simulink model "simTr"  (R2018b)
settings: Solver=FixedStepAuto  StartTime=0.0  StopTime=100  FixedStep=0.001  RelTol=1e-3
values from neighbouring files (symbols this model uses):
  dfwe1 = 0.1 * fwe1max    [script8.m]
  dt = 20    [script8.m]
  fwe2 = 0.2594    [script8.m]
  h10 = (fwe1 / a1) + h20    [script8.m]
  h20 = (fwe1 + fwe2)/a2    [script8.m]
  Lh1f1 = [A2 a1+a2]    [script8.m]
  Lh1f2 = [a1]    [script8.m]
  Lh2f1 = [a1]    [script8.m]
  Lh2f2 = [A1 a1]    [script8.m]
  M = [A1*A2 a1*A1+a2*A1+a1*A2 a1*a1+a1*a2]    [script8.m]
settings Model: Creator=wojciechkonury  LastModifiedBy=wojciechkonury

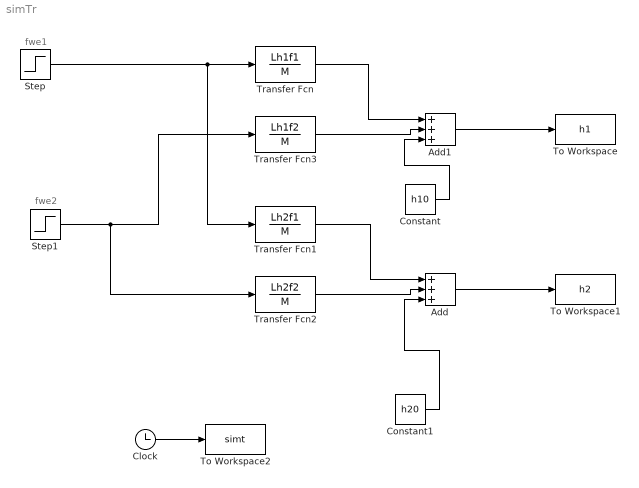
== system simTr ==
  note: fwe2
  note: fwe1
  Add : Sum  Inputs=+++
  Add1 : Sum  Inputs=+++
  Clock : Clock
  Constant : Constant  Value=h10
  Constant1 : Constant  Value=h20
  Step : Step  Time=dt  After=dfwe1  SampleTime=0
  Step1 : Step  Time=dt  After=fwe2  SampleTime=0
  To Workspace : ToWorkspace  VariableName=h1  SampleTime=-1
  To Workspace1 : ToWorkspace  VariableName=h2  SampleTime=-1
  To Workspace2 : ToWorkspace  VariableName=simt  SampleTime=-1
  Transfer Fcn : TransferFcn  Numerator=Lh1f1  Denominator=M
  Transfer Fcn1 : TransferFcn  Numerator=Lh2f1  Denominator=M
  Transfer Fcn2 : TransferFcn  Numerator=Lh2f2  Denominator=M
  Transfer Fcn3 : TransferFcn  Numerator=Lh1f2  Denominator=M
  wires:
  Step/1 -> Transfer Fcn1/1, Transfer Fcn/1
  Transfer Fcn/1 -> Add1/1
  Add1/1 -> To Workspace/1
  Add/1 -> To Workspace1/1
  Step1/1 -> Transfer Fcn2/1, Transfer Fcn3/1
  Transfer Fcn3/1 -> Add1/2
  Transfer Fcn1/1 -> Add/1
  Transfer Fcn2/1 -> Add/2
  Clock/1 -> To Workspace2/1
  Constant/1 -> Add1/3
  Constant1/1 -> Add/3
